simulink model "Linear_model"  (R2023a)
settings: Solver=VariableStepAuto  StartTime=0.0  StopTime=4  RelTol=1e-3
undefined symbols (not defined in the file): ak0, ak1, ap0, ap1, bk0, bk1, bp0, bp1, i, J_rot, Jk, K_m, Kc, kdp, Ki, kip, Kk, kpid, kpp, R_3ph, T_q
settings Model: Creator=Artem Sannikov  LastModifiedBy=Artem Sannikov

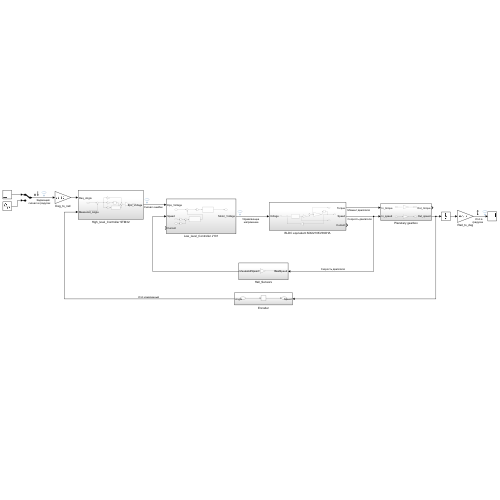
[thumbnail: Simulink's stored preview of the top-level diagram]
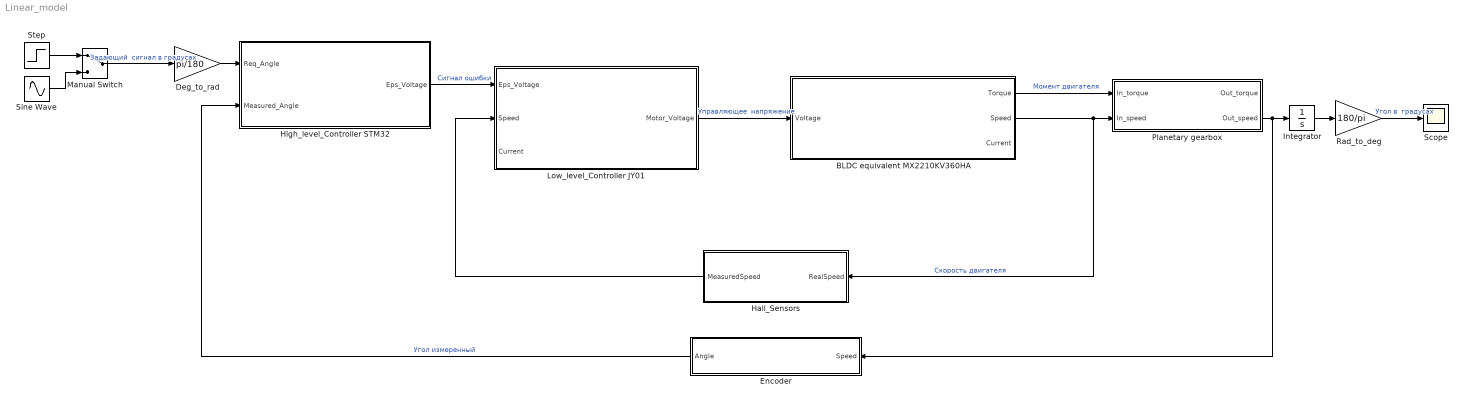
== system Linear_model ==
  BLDC equivalent MX2210KV360HA : Subsystem
  Deg_to_rad : Gain  Gain=pi/180
  Encoder : Subsystem
  Hall_Sensors : Subsystem
  High_level_Controller STM32 : Subsystem
  Integrator : Integrator
  Low_level_Controller JY01 : Subsystem
  Manual Switch : ManualSwitch
  Planetary gearbox : Subsystem
  Rad_to_deg : Gain  Gain=180/pi
  Scope : Scope
  Sine Wave : Sin  Amplitude=180  Frequency=10  SampleTime=0
  Step : Step  After=360  SampleTime=0
  wires:
  BLDC equivalent MX2210KV360HA/2(Speed) -> Planetary gearbox/2(In_speed), Hall_Sensors/1(RealSpeed)  "Скорость двигателя"
  BLDC equivalent MX2210KV360HA/1(Torque) -> Planetary gearbox/1(In_torque)  "Момент двигателя"
  Planetary gearbox/2(Out_speed) -> Integrator/1, Encoder/1(Speed)
  Hall_Sensors/1(MeasuredSpeed) -> Low_level_Controller JY01/2(Speed)
  Low_level_Controller JY01/1(Motor_Voltage) -> BLDC equivalent MX2210KV360HA/1(Voltage)  "Управляющее  напряжение"
  High_level_Controller STM32/1(Eps_Voltage) -> Low_level_Controller JY01/1(Eps_Voltage)  "Сигнал ошибки"
  Encoder/1(Angle) -> High_level_Controller STM32/2(Measured_Angle)  "Угол измеренный"
  Manual Switch/1 -> Deg_to_rad/1  "Задающий  сигнал в градусах"
  Deg_to_rad/1 -> High_level_Controller STM32/1(Req_Angle)
  Integrator/1 -> Rad_to_deg/1
  Rad_to_deg/1 -> Scope/1  "Угол в  градусах"
  Step/1 -> Manual Switch/1
  Sine Wave/1 -> Manual Switch/2

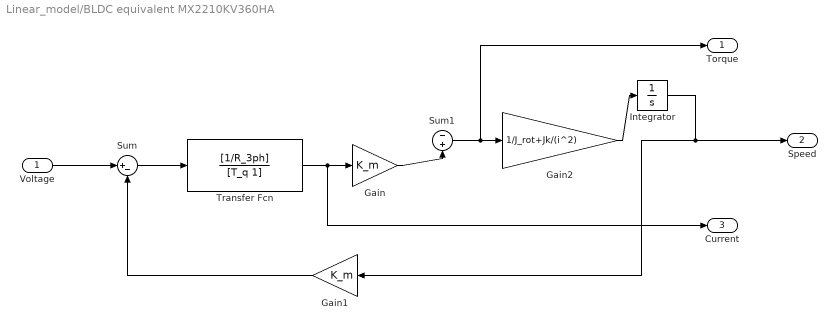
== system Linear_model/BLDC equivalent MX2210KV360HA ==
  Voltage : Inport
  Gain : Gain  Gain=K_m
  Gain1 : Gain  Gain=K_m
  Gain2 : Gain  Gain=1/J_rot+Jk/(i^2)
  Integrator : Integrator
  Sum : Sum  Inputs=|+-
  Sum1 : Sum  Inputs=-|+
  Transfer Fcn : TransferFcn  Numerator=[1/R_3ph]  Denominator=[T_q 1]
  Torque : Outport
  Speed : Outport  Port=2
  Current : Outport  Port=3
  wires:
  Voltage/1 -> Sum/1
  Sum/1 -> Transfer Fcn/1
  Transfer Fcn/1 -> Current/1, Gain/1
  Gain/1 -> Sum1/2
  Sum1/1 -> Torque/1, Gain2/1
  Gain1/1 -> Sum/2
  Integrator/1 -> Gain1/1, Speed/1
  Gain2/1 -> Integrator/1

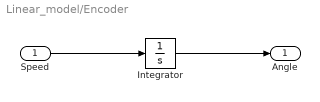
== system Linear_model/Encoder ==
  Speed : Inport
  Integrator : Integrator
  Angle : Outport
  wires:
  Speed/1 -> Integrator/1
  Integrator/1 -> Angle/1

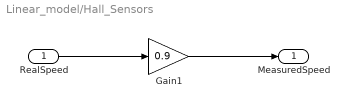
== system Linear_model/Hall_Sensors ==
  RealSpeed : Inport
  Gain1 : Gain  Gain=0.9
  MeasuredSpeed : Outport
  wires:
  RealSpeed/1 -> Gain1/1
  Gain1/1 -> MeasuredSpeed/1

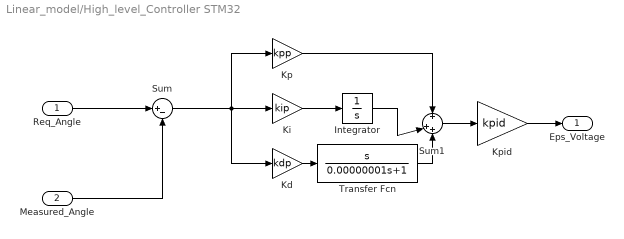
== system Linear_model/High_level_Controller STM32 ==
  Req_Angle : Inport
  Measured_Angle : Inport  Port=2
  Integrator : Integrator
  Kd : Gain  Gain=kdp
  Ki : Gain  Gain=kip
  Kp : Gain  Gain=kpp
  Kpid : Gain  Gain=kpid
  Sum : Sum  Inputs=|+-
  Sum1 : Sum  Inputs=+|++
  Transfer Fcn : TransferFcn  Numerator=[1 0]  Denominator=[0.00000001 1]
  Eps_Voltage : Outport
  wires:
  Req_Angle/1 -> Sum/1
  Measured_Angle/1 -> Sum/2
  Kpid/1 -> Eps_Voltage/1
  Ki/1 -> Integrator/1
  Integrator/1 -> Sum1/2
  Kp/1 -> Sum1/1
  Sum/1 -> Kd/1, Kp/1, Ki/1
  Sum1/1 -> Kpid/1
  Kd/1 -> Transfer Fcn/1
  Transfer Fcn/1 -> Sum1/3

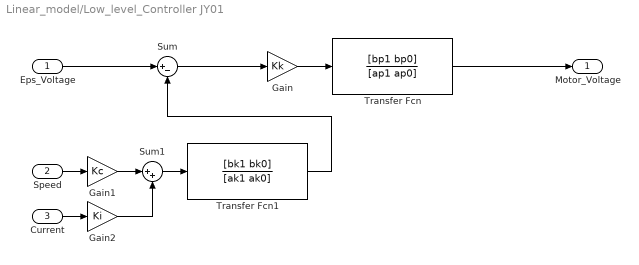
== system Linear_model/Low_level_Controller JY01 ==
  Eps_Voltage : Inport
  Speed : Inport  Port=2
  Current : Inport  Port=3
  Gain : Gain  Gain=Kk
  Gain1 : Gain  Gain=Kc
  Gain2 : Gain  Gain=Ki
  Sum : Sum  Inputs=|+-
  Sum1 : Sum  Inputs=|++
  Transfer Fcn : TransferFcn  Numerator=[bp1 bp0]  Denominator=[ap1 ap0]
  Transfer Fcn1 : TransferFcn  Numerator=[bk1 bk0]  Denominator=[ak1 ak0]
  Motor_Voltage : Outport
  wires:
  Eps_Voltage/1 -> Sum/1
  Current/1 -> Gain2/1
  Speed/1 -> Gain1/1
  Gain2/1 -> Sum1/2
  Gain1/1 -> Sum1/1
  Sum1/1 -> Transfer Fcn1/1
  Transfer Fcn1/1 -> Sum/2
  Sum/1 -> Gain/1
  Gain/1 -> Transfer Fcn/1
  Transfer Fcn/1 -> Motor_Voltage/1

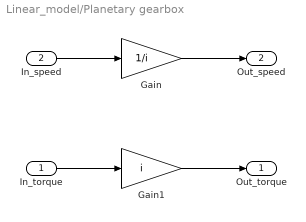
== system Linear_model/Planetary gearbox ==
  In_torque : Inport
  In_speed : Inport  Port=2
  Gain : Gain  Gain=1/i
  Gain1 : Gain  Gain=i
  Out_torque : Outport
  Out_speed : Outport  Port=2
  wires:
  In_speed/1 -> Gain/1
  Gain/1 -> Out_speed/1
  In_torque/1 -> Gain1/1
  Gain1/1 -> Out_torque/1
